simulink model "infeed_base"  (R2023b)
settings: Solver=VariableStepAuto  StartTime=0.0  StopTime=.3  MaxStep=1e-3  RelTol=1e-3  AbsTol=1e-3  EnableMultiTasking=on
values from neighbouring files (symbols this model uses):
  Ts = ts(k)    [example_MW.m]
  Un = 400    [example_MW.m]
undefined symbols (not defined in the file or in its folder): Cz, It1base, Ki_id, Ki_iq, Ki_vdc, Kp_id, Kp_iq, Kp_vdc, Le, Leq, Lk, om, Req, Rz, Tsc, Udc, Vt1base, wtbase, X_R_Le, X_R_Lk
libraries: ee_lib x15, nesl_utility x11, fl_lib x6, eeGeneralControl x4, eeTransforms x3, slpidlib x2, eeAdaptiveController x1, eePwmGeneratorTwoLevel x1, eeSinusoidalMeasurement x1
settings Model: SimulationMode=accelerator  Creator=neugebch  LastModifiedBy=neugebch
settings SolverCC: AutoScaleAbsTol=off  AlgebraicLoopSolver=TrustRegion  MaxZcPerStep=1
settings DataIOCC: LimitDataPoints=on  MaxDataPoints=10000
settings OptimizationCC: ReuseModelBlockBuffer=off  LifeSpan=inf
settings DebuggingCC: UnconnectedInputMsg=warning  UnconnectedOutputMsg=warning  UnconnectedLineMsg=warning  AllowSymbolicDim=off  SFUnexpectedBacktrackingDiag=warning  SFNoUnconditionalDefaultTransitionDiag=warning  SFExecutionAtInitializationDiag=none  ArithmeticOperatorsInVariantConditions=warning
settings ModelReferenceCC: EnableRefExpFcnMdlSchedulingChecks=on
settings SFSimCC: SimUseLocalCustomCode=off  CustomCodeUndefinedFunction=UseInterfaceOnly
settings RTWCC: RTWUseLocalCustomCode=off  DLArmComputeVersion=19.05
settings CodeAppCC: StateflowObjectComments=on
settings GRTTargetCC: TargetLangStandard=C89/C90 (ANSI)
settings ConfigComp: CovMetricSettings=dw  CovSaveCumulativeToWorkspaceVar=on  CovSaveSingleToWorkspaceVar=on  CovExternalEMLEnable=off  CovSFcnEnable=off
settings SimscapeCC: SimscapeLogType=all  SimscapeLogSimulationStatistics=on  SimscapeLogDataHistory=10000

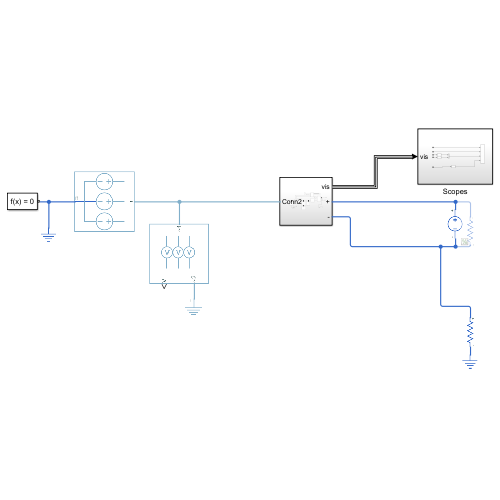
[thumbnail: Simulink's stored preview of the top-level diagram]
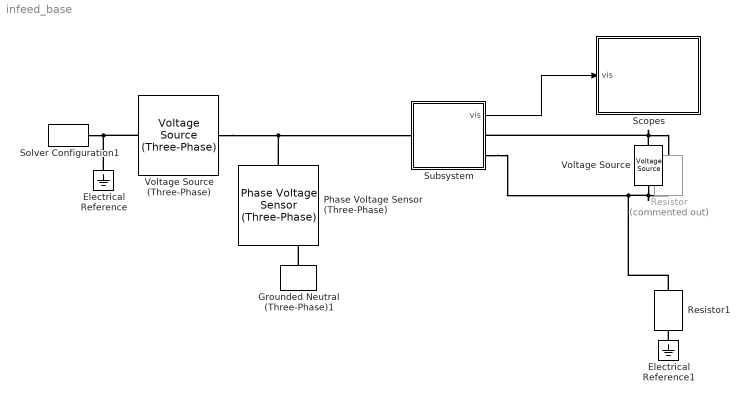
== system infeed_base ==
  Electrical Reference : fl_lib/Electrical/Electrical Elements/Electrical Reference
  Electrical Reference1 : fl_lib/Electrical/Electrical Elements/Electrical Reference
  Grounded Neutral (Three-Phase)1 : ee_lib/Connectors & References/Grounded Neutral (Three-Phase)
  Phase Voltage Sensor (Three-Phase) : ee_lib/Sensors & Transducers/Phase Voltage Sensor (Three-Phase)
  Resistor : fl_lib/Electrical/Electrical Elements/Resistor  Commented=on  R=2 Ohm  i_specify=off  i_priority=None  i=0 A  i_nominal_specify=off  i_nominal_unit=A  i_nominal_value=1  v_specify=off  v_priority=None  v=0 V  v_nominal_specify=off  v_nominal_unit=V  v_nominal_value=1
  Resistor1 : fl_lib/Electrical/Electrical Elements/Resistor  R=1e6 Ohm  i_specify=off  i_priority=None  i=0 A  i_nominal_specify=off  i_nominal_unit=A  i_nominal_value=1  v_specify=off  v_priority=None  v=0 V  v_nominal_specify=off  v_nominal_unit=V  v_nominal_value=1
  Scopes : Subsystem
  Solver Configuration1 : nesl_utility/Solver Configuration  PhysicalDomain=network_engine_domain  SubClassName=solver  LeftPortType=input  RightPortType=generic  Tones=[]  Harmonics=[]  SimulateNoise=off  Profile=off  UseLocalSampling=off  EnableSwitchedLinearOptims=on  FrequencyDomain=off  UseCCode=off  RelTol=0.001  AbsTol=1e-06  MinStep=1e-09  ToWorkspace=off  RevertToSquareIcSolve=off  NumHomotopyIterations=100  PhasorMode=off  PhasorModeNumHarmonics=1  ConsistencySolver=NEWTON_FTOL  IndexReductionMethod=DerivativeReplacement  DoDC=off  ResidualTolerance=1e-09  ConsistencyTolSource=GLOBAL  ConsistencyAbsTol=0.001  ConsistencyRelTol=0.001  ConsistencyTolFactor=0.001  UseLocalSolver=on  LocalSolverChoice=NE_PARTITIONING_ADVANCER  ResolveIndetEquations=on  FunctionEvalNumThread=1  LocalSolverSampleTime=Ts  DoFixedCost=on  MaxNonlinIter=5  MaxModeIter=2  ComputeImpulses=off  ImpulseIterations=1  LinearAlgebra=auto  LinearAlgebraNumThread=0  EquationFormulation=NE_TIME_EF  DelaysMemoryBudget=1024  AutomaticFiltering=on  FilteringTimeConstant=0.001  PartitionStorageMethod=AS_NEEDED  PartitionMemoryBudget=1024  PartitionMethod=ROBUST  MultibodyUseLocalSolver=off  MultibodyLocalSolverChoice=ODE1  MultibodyLocalSolverSampleTime=0.001
  Subsystem : Subsystem
  Voltage Source (Three-Phase) : ee_lib/Sources/Voltage Source (Three-Phase)  vline_rms=sqrt(3) * Un / sqrt(2) V  shift=0 deg  freq=fn Hz  impedance_option=1  SShortCircuit=Skv A*V  XR=X_R  R=0.01 Ohm  L=3.97e-4 H  harmonic_option=1  harmonic_orders=[5, 7, 11, 13]  harmonic_ratios=[.1, .1, .1, .1]  G_parasitic=0 1/Ohm  I_specify=off  I_priority=None  I=[0, 0, 0] A  I_nominal_specify=off  I_nominal_unit=A  I_nominal_value=1
  Voltage Source : ee_lib/Sources/Voltage Source  dc_voltage=Udc V  ac_voltage=0 V  ac_shift=0 rad  ac_frequency=fn Hz  noise_mode=ee.enum.sources.noise.Disabled  PSD=0 V^2/Hz  sample_time=1e-3 s  repeatability=ee.enum.sources.repeatability.NotRepeatable  user_seed=0  auto_seed=3499211588  i_specify=off  i_priority=None  i=0 A  i_nominal_specify=off  i_nominal_unit=A  i_nominal_value=1  v_specify=off  v_priority=None  v=0 V  v_nominal_specify=off  v_nominal_unit=V  v_nominal_value=1
  wires:
  Subsystem/1(vis) -> Scopes/1(vis)
  connections:
  Electrical Reference/LConn1 -- Solver Configuration1/RConn1 -- Voltage Source (Three-Phase)/LConn1
  Grounded Neutral (Three-Phase)1/LConn1 -- Phase Voltage Sensor (Three-Phase)/RConn2
  Voltage Source/RConn1 -- Resistor1/LConn1 -- Subsystem/RConn2 -- Resistor/RConn1
  Electrical Reference1/LConn1 -- Resistor1/RConn1
  Voltage Source/LConn1 -- Subsystem/RConn1 -- Resistor/LConn1
  Voltage Source (Three-Phase)/RConn1 -- Phase Voltage Sensor (Three-Phase)/LConn1 -- Subsystem/LConn1

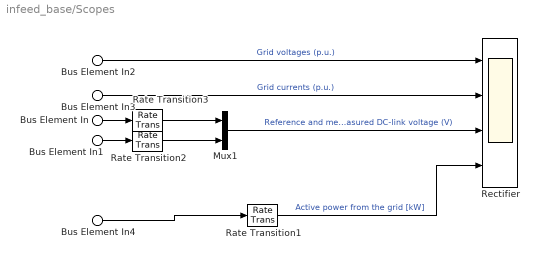
== system infeed_base/Scopes ==
  Bus Element In : Inport  PortName=vis  Element=VdcRef
  Bus Element In1 : Inport  PortName=vis  Element=VdcF
  Bus Element In2 : Inport  PortName=vis  Element=VgABC
  Bus Element In3 : Inport  PortName=vis  Element=IgABC
  Bus Element In4 : Inport  PortName=vis  Element=Pt
  Mux1 : Mux  Inputs=2
  Rate Transition1 : RateTransition
  Rate Transition2 : RateTransition
  Rate Transition3 : RateTransition
  Rectifier : Scope  NumInputPorts=4
  wires:
  Rate Transition2/1 -> Mux1/2
  Bus Element In/1 -> Rate Transition3/1
  Mux1/1 -> Rectifier/3  "Reference and measured DC-link voltage (V)"
  Bus Element In4/1 -> Rate Transition1/1
  Bus Element In2/1 -> Rectifier/1  "Grid voltages (p.u.)"
  Bus Element In3/1 -> Rectifier/2  "Grid currents (p.u.)"
  Rate Transition1/1 -> Rectifier/4  "Active power from the grid [kW]"
  Bus Element In1/1 -> Rate Transition2/1
  Rate Transition3/1 -> Mux1/1

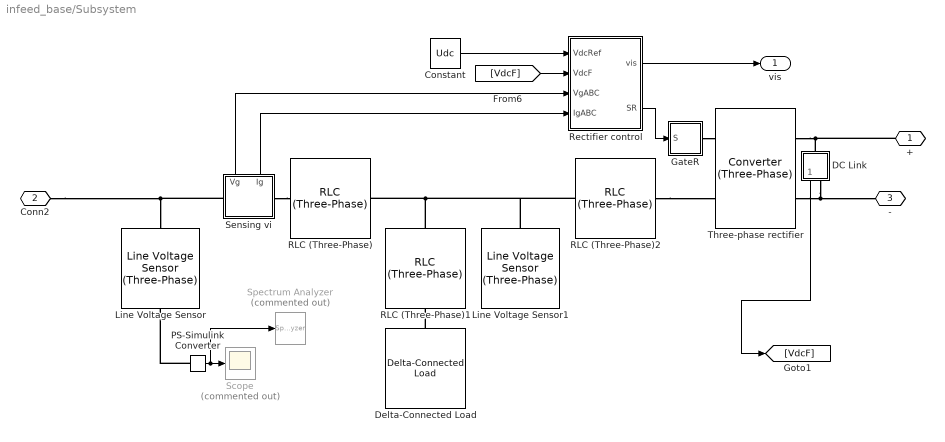
== system infeed_base/Subsystem ==
  Constant : Constant  Value=Udc
  DC Link : Subsystem
  Delta-Connected Load : ee_lib/Passive/RLC Assemblies/Delta-Connected Load  parameterization=ee.enum.rlc.parameterization.direct  component_structure=ee.enum.rlc.structure.C  component_structure_PQ=ee.enum.rlc.structure.SeriesRC  R=1 Ohm  L=1e-3 H  C=Cz F  VRated=24e3 V  FRated=60 Hz  P=1e3 W  Qpos=1e2 A*V  Qneg=-1e2 A*V  R_parasitic=0 Ohm  G_parasitic=0 1/Ohm  R_parasitic_PQ=0 Ohm  G_parasitic_PQ=0 1/Ohm  Vmag0=24e3 V  Vang0=0 deg  Freq0=60 Hz  IL_specify=off  IL_priority=High  IL=[0, 0, 0] A  IL_nominal_specify=off  IL_nominal_unit=A  IL_nominal_value=1  VC_specify=off  VC_priority=High  VC=[0, 0, 0] V  VC_nominal_specify=off  VC_nominal_unit=V  VC_nominal_value=1
      settings: InternalSimscapePortConfiguration="{\"Bottom\":[],\"Left\":[{\"id\":\"N\",\"label\":\"~\",\"type\":\"foundation.electrical.three_phase\"}],\"Right\":[],\"Top\":[]}"
  GateR : Subsystem
  Line Voltage Sensor : ee_lib/Sensors & Transducers/Line Voltage Sensor (Three-Phase)
  Line Voltage Sensor1 : ee_lib/Sensors & Transducers/Line Voltage Sensor (Three-Phase)
  PS-Simulink Converter : nesl_utility/PS-Simulink Converter  PhysicalDomain=network_engine_domain  SubClassName=ps_output  LeftPortType=input  RightPortType=output  PseudoPeriodic=off  Frequencies=[]  VectorFormat=inherit  Unit=inherit  AffineConversion=off
  RLC (Three-Phase) : ee_lib/Passive/RLC Assemblies/RLC (Three-Phase)  component_structure=ee.enum.rlc.structure.SeriesRL  R=Le*om/X_R_Le Ohm  L=Le H  C=1e-6 F  R_parasitic=0 Ohm  G_parasitic=0 1/Ohm  IL_specify=off  IL_priority=High  IL=[0, 0, 0] A  IL_nominal_specify=off  IL_nominal_unit=A  IL_nominal_value=1  VC_specify=off  VC_priority=High  VC=[0, 0, 0] V  VC_nominal_specify=off  VC_nominal_unit=V  VC_nominal_value=1
      settings: InternalSimscapePortConfiguration="{\"Bottom\":[],\"Left\":[{\"id\":\"N1\",\"label\":\"~1\",\"type\":\"foundation.electrical.three_phase\"}],\"Right\":[{\"id\":\"N2\",\"label\":\"~2\",\"type\":\"foundation.electrical.three_phase\"}],\"Top\":[]}"
  RLC (Three-Phase)1 : ee_lib/Passive/RLC Assemblies/RLC (Three-Phase)  component_structure=ee.enum.rlc.structure.R  R=Rz Ohm  L=1e-3 H  C=1e-6 F  R_parasitic=0 Ohm  G_parasitic=0 1/Ohm  IL_specify=off  IL_priority=High  IL=[0, 0, 0] A  IL_nominal_specify=off  IL_nominal_unit=A  IL_nominal_value=1  VC_specify=off  VC_priority=High  VC=[0, 0, 0] V  VC_nominal_specify=off  VC_nominal_unit=V  VC_nominal_value=1
      settings: InternalSimscapePortConfiguration="{\"Bottom\":[],\"Left\":[{\"id\":\"N1\",\"label\":\"~1\",\"type\":\"foundation.electrical.three_phase\"}],\"Right\":[{\"id\":\"N2\",\"label\":\"~2\",\"type\":\"foundation.electrical.three_phase\"}],\"Top\":[]}"
  RLC (Three-Phase)2 : ee_lib/Passive/RLC Assemblies/RLC (Three-Phase)  component_structure=ee.enum.rlc.structure.SeriesRL  R=Lk*om/X_R_Lk Ohm  L=Lk H  C=1e-6 F  R_parasitic=0 Ohm  G_parasitic=0 1/Ohm  IL_specify=off  IL_priority=High  IL=[0, 0, 0] A  IL_nominal_specify=off  IL_nominal_unit=A  IL_nominal_value=1  VC_specify=off  VC_priority=High  VC=[0, 0, 0] V  VC_nominal_specify=off  VC_nominal_unit=V  VC_nominal_value=1
      settings: InternalSimscapePortConfiguration="{\"Bottom\":[],\"Left\":[{\"id\":\"N1\",\"label\":\"~1\",\"type\":\"foundation.electrical.three_phase\"}],\"Right\":[{\"id\":\"N2\",\"label\":\"~2\",\"type\":\"foundation.electrical.three_phase\"}],\"Top\":[]}"
  Rectifier control : Subsystem
  Scope : Scope  Commented=on
  Sensing vi : Subsystem
      settings: PortSchema="{\"entries\":[{\"content\":{\"sides\":[{\"content\":{\"connectorIds\":[\"LConn1\"]},\"type\":\"ConnectorPlacement.EquallySpacedRectSide\",\"uuid\":\"c5057f2e-2c18-4118-b873-a75143a124e4\"},{\"content\":{\"connectorIds\":[\"RConn1\"],\"side\":\"RIGHT\"},\"type\":\"ConnectorPlacement.EquallySpacedRectSide\",\"uuid\":\"847dbac9-66f5-462a-b095-b42c8738b9ce\"},{\"content\":{\"connectorIds\":[\"Out1\",\"Out2\"],\"side\":\"TOP\"},\"type\":\"ConnectorPlacement.EquallySpacedRectSide\",\"uuid\":\"1cd52aa7-c39c-45ef-b799-a348546c5bc9\"}]},\"type\":\"ConnectorPlacement.EquallySpacedConnector\",\"uuid\":\"7d89bf63-b784-4419-8d3e-10ce7abb2518\"}],\"packageUris\":[\"http://schema.mathworks.com/mf0/Connector/R2020b\"],\"version\":\"1.0\"}"
  Spectrum Analyzer : SpectrumAnalyzer  Commented=on  WindowPosition=[1 31 1920 973]  Method=Welch  SampleRate=1000000  PlotAsTwoSidedSpectrum=off  AxesScaling=Manual  Span=500000  CenterFrequency=250000  StartFrequency=0  StopFrequency=500000  RBWSource=Property  RBW=5  Window=Rectangular  AveragingMethod=Exponential  YLimits=[-2.9752431145922511035,92.887308708132081847]
  Three-phase rectifier : ee_lib/Semiconductors & Converters/Converters/Converter (Three-Phase)  port_option=ee.enum.threePhasePort.composite  device_type=ee.enum.converters.switchingdevice.igbt  K=0  Vf=0.8 V  Ron=0.001 Ohm  Rds=0.001 Ohm  Goff=1e-5 1/Ohm  Vgt=1 V  Vgt_off=-1 V  Ih=1 A  Vth=0.5 V  diode_param=ee.enum.converters.protectiondiode.nodynamics  diode_Vf=0.8 V  diode_Ron=0.001 Ohm  diode_Goff=1e-5 1/Ohm  diode_C=50 nF  diode_iRM=-235 A  diode_iF=300 A  diode_idot=-50 A/us  diode_trr_param=ee.enum.converters.diodetrr.trr_factor  diode_trr_factor=3  diode_trr=15 us  diode_Qrr=1.5e+3 s*uA  snubber_type=ee.enum.converters.snubber.exclude  Cs=1e-5 F  Rs=1e-3 Ohm
  + : PMIOPort  Side=Right
  Conn2 : PMIOPort  Port=2  Side=Left
  - : PMIOPort  Port=3  Side=Right
  vis : Outport
  wires:
  Sensing vi/2(Ig) -> Rectifier control/4(IgABC)
  Rectifier control/1(vis) -> vis/1
  PS-Simulink Converter/1 -> Spectrum Analyzer/1, Scope/1
  Sensing vi/1(Vg) -> Rectifier control/3(VgABC)
  [VdcF] -> Rectifier control/2(VdcF)
  Rectifier control/2(SR) -> GateR/1(S)
  Constant/1 -> Rectifier control/1(VdcRef)
  DC Link/1(vdcF) -> [VdcF]
  connections:
  RLC (Three-Phase)1/LConn1 -- Line Voltage Sensor1/LConn1 -- RLC (Three-Phase)2/LConn1 -- RLC (Three-Phase)/RConn1
  PS-Simulink Converter/LConn1 -- Line Voltage Sensor/RConn1
  RLC (Three-Phase)2/RConn1 -- Three-phase rectifier/LConn2
  Sensing vi/LConn1 -- Conn2/RConn1 -- Line Voltage Sensor/LConn1
  Three-phase rectifier/RConn1 -- +/RConn1 -- DC Link/LConn1
  Delta-Connected Load/LConn1 -- RLC (Three-Phase)1/RConn1
  GateR/RConn1 -- Three-phase rectifier/LConn1
  DC Link/RConn1 -- -/RConn1 -- Three-phase rectifier/RConn2
  Sensing vi/RConn1 -- RLC (Three-Phase)/LConn1

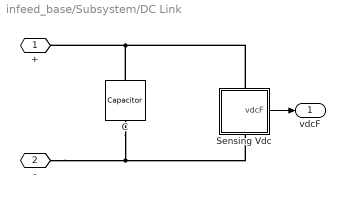
== system infeed_base/Subsystem/DC Link ==
  C : fl_lib/Electrical/Electrical Elements/Capacitor  c=500e-6; F  r=2e-3 Ohm  g=0 1/Ohm  i_specify=off  i_priority=None  i=0 A  i_nominal_specify=off  i_nominal_unit=A  i_nominal_value=1  v_specify=off  v_priority=None  v=0 V  v_nominal_specify=off  v_nominal_unit=V  v_nominal_value=1  vc_specify=on  vc_priority=None  vc=0 V  vc_nominal_specify=off  vc_nominal_unit=V  vc_nominal_value=1
  Sensing Vdc : Subsystem
      settings: PortSchema="{\"entries\":[{\"content\":{\"sides\":[{\"content\":{\"connectorIds\":[\"LConn1\"]},\"type\":\"ConnectorPlacement.EquallySpacedRectSide\",\"uuid\":\"0c76379d-baff-4140-87e0-7680e80a3e64\"},{\"content\":{\"connectorIds\":[\"RConn1\"],\"side\":\"RIGHT\"},\"type\":\"ConnectorPlacement.EquallySpacedRectSide\",\"uuid\":\"435fa78d-19d1-48b9-8f1c-afd8cf746df8\"},{\"content\":{\"connectorIds\":[],\"side\":\"TOP\"},\"type\":\"ConnectorPlacement.EquallySpacedRectSide\",\"uuid\":\"64f7027d-3f1c-43c6-9f97-24bcd914447a\"},{\"content\":{\"connectorIds\":[\"Out1\"],\"side\":\"BOTTOM\"},\"type\":\"ConnectorPlacement.EquallySpacedRectSide\",\"uuid\":\"c8d3e8f7-8819-4adf-938e-d95e3be67703\"}]},\"type\":\"ConnectorPlacement.EquallySpacedConnector\",\"uuid\":\"559fa4aa-2e9f-4f72-acfb-6b72122ee549\"}],\"packageUris\":[\"http://schema.mathworks.com/mf0/Connector/R2020b\"],\"version\":\"1.0\"}"
  + : PMIOPort  Side=Left
  - : PMIOPort  Port=2  Side=Right
  vdcF : Outport
  wires:
  Sensing Vdc/1(vdcF) -> vdcF/1
  connections:
  -/RConn1 -- C/RConn1 -- Sensing Vdc/RConn1
  C/LConn1 -- Sensing Vdc/LConn1 -- +/RConn1

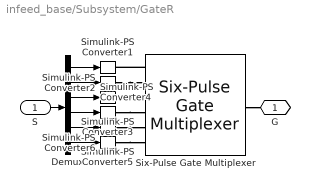
== system infeed_base/Subsystem/GateR ==
  S : Inport
  Demux : Demux  Outputs=6
  Simulink-PS Converter{1..6} (6 alike) : nesl_utility/Simulink-PS Converter  PhysicalDomain=network_engine_domain  SubClassName=ps_input  LeftPortType=input  RightPortType=output  PseudoPeriodic=off  Frequencies=[]  NoiseDistribution=none  NoiseParameters=[]  Unit=1  AffineConversion=off  FilteringAndDerivatives=zero  SimscapeFilterOrder=1  InputFilterTimeConstant=0.001  UdotUserProvided=1
  Six-Pulse Gate Multiplexer : ee_lib/Semiconductors & Converters/Converters/Six-Pulse Gate Multiplexer  port_option=ee.enum.controlport.ps
  G : PMIOPort  Side=Right
  wires:
  Demux/4 -> Simulink-PS Converter4/1
  Demux/1 -> Simulink-PS Converter1/1
  Demux/2 -> Simulink-PS Converter2/1
  S/1 -> Demux/1
  Demux/5 -> Simulink-PS Converter5/1
  Demux/6 -> Simulink-PS Converter6/1
  Demux/3 -> Simulink-PS Converter3/1
  connections:
  Simulink-PS Converter4/RConn1 -- Six-Pulse Gate Multiplexer/LConn4
  Simulink-PS Converter2/RConn1 -- Six-Pulse Gate Multiplexer/LConn2
  Simulink-PS Converter3/RConn1 -- Six-Pulse Gate Multiplexer/LConn3
  Simulink-PS Converter6/RConn1 -- Six-Pulse Gate Multiplexer/LConn6
  Simulink-PS Converter5/RConn1 -- Six-Pulse Gate Multiplexer/LConn5
  Six-Pulse Gate Multiplexer/LConn1 -- Simulink-PS Converter1/RConn1
  Six-Pulse Gate Multiplexer/RConn1 -- G/RConn1

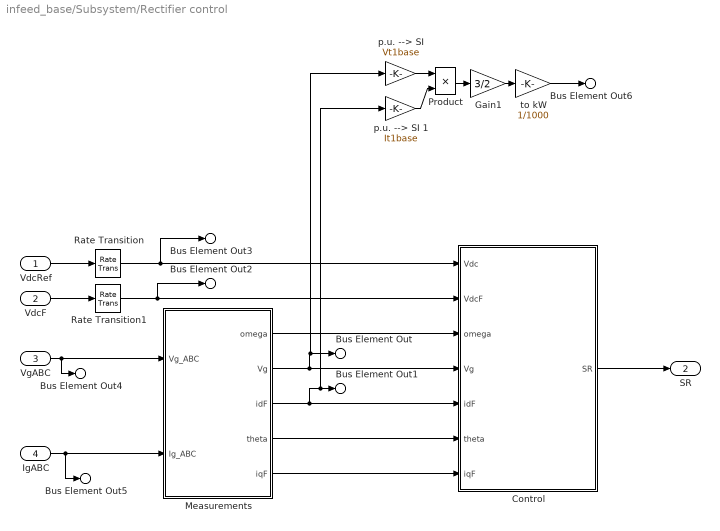
== system infeed_base/Subsystem/Rectifier control ==
  VdcRef : Inport
  VdcF : Inport  Port=2
  VgABC : Inport  Port=3
  IgABC : Inport  Port=4
  Control : Subsystem
  Gain1 : Gain  Gain=3/2
  Measurements : Subsystem
  Product : Product
  Rate Transition : RateTransition
  Rate Transition1 : RateTransition
  p.u. --> SI : Gain  Gain=Vt1base
  p.u. --> SI 1 : Gain  Gain=It1base
  to kW : Gain  Gain=1/1000
  Bus Element Out : Outport  PortName=vis  Element=Vg
  Bus Element Out1 : Outport  PortName=vis  Element=idF
  Bus Element Out2 : Outport  PortName=vis  Element=VdcF
  Bus Element Out3 : Outport  PortName=vis  Element=VdcRef
  Bus Element Out4 : Outport  PortName=vis  Element=VgABC
  Bus Element Out5 : Outport  PortName=vis  Element=IgABC
  Bus Element Out6 : Outport  PortName=vis  Element=Pt
  SR : Outport  Port=2  VectorParamsAs1DForOutWhenUnconnected=off
  wires:
  VdcRef/1 -> Rate Transition/1
  VdcF/1 -> Rate Transition1/1
  VgABC/1 -> Bus Element Out4/1, Measurements/1(Vg_ABC)
  IgABC/1 -> Bus Element Out5/1, Measurements/2(Ig_ABC)
  Measurements/1(omega) -> Control/3(omega)
  Measurements/4(theta) -> Control/6(theta)
  Measurements/5(iqF) -> Control/7(iqF)
  Control/1(SR) -> SR/1
  Rate Transition/1 -> Bus Element Out3/1, Control/1(Vdc)
  Rate Transition1/1 -> Bus Element Out2/1, Control/2(VdcF)
  Measurements/2(Vg) -> p.u. --> SI/1, Bus Element Out/1, Control/4(Vg)
  p.u. --> SI 1/1 -> Product/2
  p.u. --> SI/1 -> Product/1
  Gain1/1 -> to kW/1
  Product/1 -> Gain1/1
  Measurements/3(idF) -> p.u. --> SI 1/1, Bus Element Out1/1, Control/5(idF)
  to kW/1 -> Bus Element Out6/1

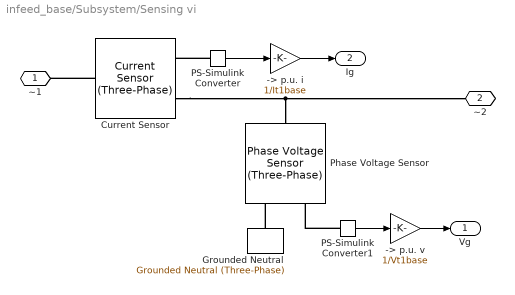
== system infeed_base/Subsystem/Sensing vi ==
  -> p.u. i : Gain  Gain=1/It1base
  -> p.u. v : Gain  Gain=1/Vt1base
  Current Sensor : ee_lib/Sensors & Transducers/Current Sensor (Three-Phase)
  Grounded Neutral : ee_lib/Connectors & References/Grounded Neutral (Three-Phase)
  PS-Simulink Converter : nesl_utility/PS-Simulink Converter  PhysicalDomain=network_engine_domain  SubClassName=ps_output  LeftPortType=input  RightPortType=output  PseudoPeriodic=off  Frequencies=[]  VectorFormat=1-D array  Unit=1  AffineConversion=off
  PS-Simulink Converter1 : nesl_utility/PS-Simulink Converter  PhysicalDomain=network_engine_domain  SubClassName=ps_output  LeftPortType=input  RightPortType=output  PseudoPeriodic=off  Frequencies=[]  VectorFormat=1-D array  Unit=1  AffineConversion=off
  Phase Voltage Sensor : ee_lib/Sensors & Transducers/Phase Voltage Sensor (Three-Phase)
  ~1 : PMIOPort  Side=Left
  ~2 : PMIOPort  Port=2  Side=Right
  Vg : Outport
  Ig : Outport  Port=2
  wires:
  -> p.u. i/1 -> Ig/1
  PS-Simulink Converter1/1 -> -> p.u. v/1
  PS-Simulink Converter/1 -> -> p.u. i/1
  -> p.u. v/1 -> Vg/1
  connections:
  PS-Simulink Converter1/LConn1 -- Phase Voltage Sensor/RConn1
  Current Sensor/RConn2 -- Phase Voltage Sensor/LConn1 -- ~2/RConn1
  PS-Simulink Converter/LConn1 -- Current Sensor/RConn1
  Grounded Neutral/LConn1 -- Phase Voltage Sensor/RConn2
  Current Sensor/LConn1 -- ~1/RConn1

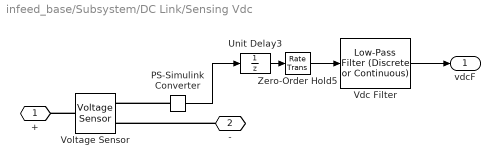
== system infeed_base/Subsystem/DC Link/Sensing Vdc ==
  PS-Simulink Converter : nesl_utility/PS-Simulink Converter  PhysicalDomain=network_engine_domain  SubClassName=ps_output  LeftPortType=input  RightPortType=output  PseudoPeriodic=off  Frequencies=[]  VectorFormat=1-D array  Unit=1  AffineConversion=off
  Unit Delay3 : UnitDelay  SampleTime=Ts  HasFrameUpgradeWarning=on
  Vdc Filter : eeGeneralControl/Low-Pass Filter (Discrete or Continuous)  K=1  T=1e-3  B=inf  A=-inf  init_option=Inherited from block input  x0=0  Ts=Tsc
  Voltage Sensor : fl_lib/Electrical/Electrical Sensors/Voltage Sensor
  Zero-Order Hold5 : RateTransition  OutPortSampleTime=5e-05
  + : PMIOPort  Side=Left
  - : PMIOPort  Port=2  Side=Right
  vdcF : Outport
  wires:
  Unit Delay3/1 -> Zero-Order Hold5/1
  Zero-Order Hold5/1 -> Vdc Filter/1
  Vdc Filter/1 -> vdcF/1
  PS-Simulink Converter/1 -> Unit Delay3/1
  connections:
  -/RConn1 -- Voltage Sensor/RConn2
  Voltage Sensor/LConn1 -- +/RConn1
  PS-Simulink Converter/LConn1 -- Voltage Sensor/RConn1

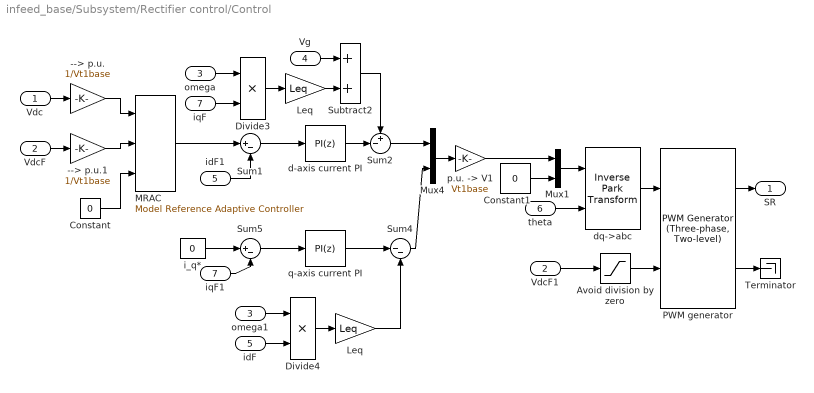
== system infeed_base/Subsystem/Rectifier control/Control ==
  Vdc : Inport
  VdcF : Inport  Port=2
  omega : Inport  Port=3
  Vg : Inport  Port=4
  idF : Inport  Port=5
  theta : Inport  Port=6
  iqF : Inport  Port=7
  --> p.u. : Gain  Gain=1/Vt1base
  --> p.u.1 : Gain  Gain=1/Vt1base
  Avoid division by zero : Saturate  UpperLimit=1e6  LowerLimit=10
  Constant : Constant  Value=0
  Constant1 : Constant  Value=0  SampleTime=Tsc
  Divide3 : Product  Inputs=**
  Divide4 : Product  Inputs=**
  Leq : Gain  Gain=Leq
  "Leq " : Gain  Gain=Leq
  MRAC : eeAdaptiveController/Model Reference Adaptive Controller  Kp=Kp_vdc  Ki=Ki_vdc  Kd=0  Kaw=1000  UseFilter=off  N=100  up=5  lo=-5  Ts=Tsc  TfType=Discrete-time  numd=numd  dend=dend  numc=[1 1]  denc=[1 2 1]  Tsd=0.01  gamma=0.8
  Mux1 : Mux  Inputs=2
  Mux4 : Mux  Inputs=2
  PWM generator : eePwmGeneratorTwoLevel/PWM Generator (Three-phase, Two-level)  PWMMode=Continuous PWM (CPWM)  CPWMMode=SVM: space vector modulation  DPWMMode=60 DPWM: 60 degree discontinuous PWM  fsw=fsw  Ts=Ts
  Subtract2 : Sum
  Sum1 : Sum  Inputs=|+-
  Sum2 : Sum  Inputs=+-|
  Sum4 : Sum  Inputs=|--
  Sum5 : Sum  Inputs=|+-
  Terminator : Terminator
  VdcF1 : InportShadow  Port=2
  d-axis current PI : slpidlib/PID Controller  Controller=PI  Form=Parallel  TimeDomain=Discrete-time  UseExternalTs=off  SampleTime=Tsc  IntegratorMethod=Forward Euler  FilterMethod=Forward Euler  ControllerParametersSource=internal  P=Kp_id  I=Ki_id  UseKiTs=off  D=0  N=100  UseFilter=on  TunerSelectOption=Transfer Function Based (PID Tuner App)  InitialConditionSource=internal  InitialConditionForIntegrator=0  InitialConditionForFilter=0  DifferentiatorICPrevScaledInput=0  ExternalReset=none  TrackingMode=off  Kt=1  LimitOutput=on  SatLimitsSource=internal  UpperSaturationLimit=Req*1*10  LowerSaturationLimit=-Req*1*10  LinearizeAsGain=on  AntiWindupMode=back-calculation  Kb=1000  LimitIntegrator=off  UpperIntegratorSaturationLimit=inf  LowerIntegratorSaturationLimit=-inf  POutMin=[]  POutMax=[]  IOutMin=[]  IOutMax=[]  DOutMin=[]  DOutMax=[]  NOutMin=[]  NOutMax=[]  SumOutMin=[]  SumOutMax=[]  SaturationOutMin=[]  SaturationOutMax=[]  PParamMin=[]  PParamMax=[]  IParamMin=[]  IParamMax=[]  DParamMin=[]  DParamMax=[]  NParamMin=[]  NParamMax=[]  KbParamMin=[]  KbParamMax=[]  KtParamMin=[]  KtParamMax=[]  KbOutMin=[]  KbOutMax=[]  KtOutMin=[]  KtOutMax=[]  IntegratorOutMin=[]  IntegratorOutMax=[]  FilterOutMin=[]  FilterOutMax=[]  SumI1OutMin=[]  SumI1OutMax=[]  SumI2OutMin=[]  SumI2OutMax=[]  SumI3OutMin=[]  SumI3OutMax=[]  SumI4OutMin=[]  SumI4OutMax=[]  SumDOutMin=[]  SumDOutMax=[]  DifferentiatorOutMin=[]  DifferentiatorOutMax=[]  FilterDiffOutCoefMin=[]  FilterDiffOutCoefMax=[]  ReciprocalOutMin=[]  ReciprocalOutMax=[]  SumDenOutMin=[]  SumDenOutMax=[]  SumNumOutMin=[]  SumNumOutMax=[]  DivideOutMin=[]  DivideOutMax=[]  UdiffTsProdOutMin=[]  UdiffTsProdOutMax=[]  NTsProdOutMin=[]  NTsProdOutMax=[]  UintegralTsProdOutMin=[]  UintegralTsProdOutMax=[]  UngainTsProdOutMin=[]  UngainTsProdOutMax=[]  ClampingZeroOutDataTypeStr=Inherit: Inherit via back propagation  ClampingZeroOutMin=[]  ClampingZeroOutMax=[]  FilterDenConstantOutDataTypeStr=Inherit: Inherit via back propagation  FilterDenConstantOutMin=[]  FilterDenConstantOutMax=[]  PCopyOutDataTypeStr=Inherit: Inherit via back propagation  PCopyOutMin=[]  PCopyOutMax=[]  NCopyOutDataTypeStr=Inherit: Inherit via back propagation  NCopyOutMin=[]  NCopyOutMax=[]  IntegratorContinuousStateAttributes=''  IntegratorStateMustResolveToSignalObject=off  IntegratorRTWStateStorageClass=Auto  FilterContinuousStateAttributes=''  FilterStateMustResolveToSignalObject=off  FilterRTWStateStorageClass=Auto  ParallelPVariant=InternalParameters  IdealPVariant=Disabled  IVariant=InternalParameters  DVariant=Disabled  IntegratorVariant=Discrete  SatVariant=Enabled  AWVariant=BackCalculation  PCopyVariant=Disabled  TRVariant=Disabled  FdbkBlocksVariant=Forward  IdealPFdbkVariant=Disabled  SatFdbkVariant=Disabled  DerivativeFilterVariant=Disabled  NVariant=Disabled  NCopyVariant=Disabled_SignalSpec  FilterICVariant=Disabled  IntegratorICVariant=InternalICs  ExternalResetVariant=Disabled  TRSumVariant=Passthrough  SumFdbkVariant=Disabled  SumVariant=Sum_PI  TsampFilterVariant=InternalTs  TsampNgainVariant=Passthrough  TsampIntegralVariant=Disabled_SignalSpec  ExternalSaturationOutDataTypeStr=Inherit: Same as second input
  dq->abc : eeTransforms/Inverse Park Transform  AxisAlignment=Q-axis  PowerInvariant=off
  i_q* : Constant  Value=0
  idF1 : InportShadow  Port=5
  iqF1 : InportShadow  Port=7
  omega1 : InportShadow  Port=3
  "p.u. -> V1" : Gain  Gain=Vt1base
  q-axis current PI : slpidlib/PID Controller  Controller=PI  Form=Parallel  TimeDomain=Discrete-time  UseExternalTs=off  SampleTime=Tsc  IntegratorMethod=Forward Euler  FilterMethod=Forward Euler  ControllerParametersSource=internal  P=Kp_iq  I=Ki_iq  UseKiTs=off  D=0  N=100  UseFilter=on  TunerSelectOption=Transfer Function Based (PID Tuner App)  InitialConditionSource=internal  InitialConditionForIntegrator=0  InitialConditionForFilter=0  DifferentiatorICPrevScaledInput=0  ExternalReset=none  TrackingMode=off  Kt=1  LimitOutput=on  SatLimitsSource=internal  UpperSaturationLimit=Req*1*10  LowerSaturationLimit=-Req*1*10  LinearizeAsGain=on  AntiWindupMode=back-calculation  Kb=1000  LimitIntegrator=off  UpperIntegratorSaturationLimit=inf  LowerIntegratorSaturationLimit=-inf  POutMin=[]  POutMax=[]  IOutMin=[]  IOutMax=[]  DOutMin=[]  DOutMax=[]  NOutMin=[]  NOutMax=[]  SumOutMin=[]  SumOutMax=[]  SaturationOutMin=[]  SaturationOutMax=[]  PParamMin=[]  PParamMax=[]  IParamMin=[]  IParamMax=[]  DParamMin=[]  DParamMax=[]  NParamMin=[]  NParamMax=[]  KbParamMin=[]  KbParamMax=[]  KtParamMin=[]  KtParamMax=[]  KbOutMin=[]  KbOutMax=[]  KtOutMin=[]  KtOutMax=[]  IntegratorOutMin=[]  IntegratorOutMax=[]  FilterOutMin=[]  FilterOutMax=[]  SumI1OutMin=[]  SumI1OutMax=[]  SumI2OutMin=[]  SumI2OutMax=[]  SumI3OutMin=[]  SumI3OutMax=[]  SumI4OutMin=[]  SumI4OutMax=[]  SumDOutMin=[]  SumDOutMax=[]  DifferentiatorOutMin=[]  DifferentiatorOutMax=[]  FilterDiffOutCoefMin=[]  FilterDiffOutCoefMax=[]  ReciprocalOutMin=[]  ReciprocalOutMax=[]  SumDenOutMin=[]  SumDenOutMax=[]  SumNumOutMin=[]  SumNumOutMax=[]  DivideOutMin=[]  DivideOutMax=[]  UdiffTsProdOutMin=[]  UdiffTsProdOutMax=[]  NTsProdOutMin=[]  NTsProdOutMax=[]  UintegralTsProdOutMin=[]  UintegralTsProdOutMax=[]  UngainTsProdOutMin=[]  UngainTsProdOutMax=[]  ClampingZeroOutDataTypeStr=Inherit: Inherit via back propagation  ClampingZeroOutMin=[]  ClampingZeroOutMax=[]  FilterDenConstantOutDataTypeStr=Inherit: Inherit via back propagation  FilterDenConstantOutMin=[]  FilterDenConstantOutMax=[]  PCopyOutDataTypeStr=Inherit: Inherit via back propagation  PCopyOutMin=[]  PCopyOutMax=[]  NCopyOutDataTypeStr=Inherit: Inherit via back propagation  NCopyOutMin=[]  NCopyOutMax=[]  IntegratorContinuousStateAttributes=''  IntegratorStateMustResolveToSignalObject=off  IntegratorRTWStateStorageClass=Auto  FilterContinuousStateAttributes=''  FilterStateMustResolveToSignalObject=off  FilterRTWStateStorageClass=Auto  ParallelPVariant=InternalParameters  IdealPVariant=Disabled  IVariant=InternalParameters  DVariant=Disabled  IntegratorVariant=Discrete  SatVariant=Enabled  AWVariant=BackCalculation  PCopyVariant=Disabled  TRVariant=Disabled  FdbkBlocksVariant=Forward  IdealPFdbkVariant=Disabled  SatFdbkVariant=Disabled  DerivativeFilterVariant=Disabled  NVariant=Disabled  NCopyVariant=Disabled_SignalSpec  FilterICVariant=Disabled  IntegratorICVariant=InternalICs  ExternalResetVariant=Disabled  TRSumVariant=Passthrough  SumFdbkVariant=Disabled  SumVariant=Sum_PI  TsampFilterVariant=InternalTs  TsampNgainVariant=Passthrough  TsampIntegralVariant=Disabled_SignalSpec  ExternalSaturationOutDataTypeStr=Inherit: Same as second input
  SR : Outport  VectorParamsAs1DForOutWhenUnconnected=off
  wires:
  Sum5/1 -> q-axis current PI/1
  theta/1 -> dq->abc/2
  Sum4/1 -> Mux4/2
  Subtract2/1 -> Sum2/1
  Sum2/1 -> Mux4/1
  Sum1/1 -> d-axis current PI/1
  Avoid division by zero/1 -> PWM generator/2
  Divide4/1 -> "Leq "/1
  Leq/1 -> Subtract2/2
  i_q*/1 -> Sum5/1
  PWM generator/1 -> SR/1
  omega/1 -> Divide3/1
  q-axis current PI/1 -> Sum4/1
  Mux4/1 -> "p.u. -> V1"/1
  Divide3/1 -> Leq/1
  Mux1/1 -> dq->abc/1
  Constant1/1 -> Mux1/2
  "Leq "/1 -> Sum4/2
  idF/1 -> Divide4/2
  PWM generator/2 -> Terminator/1
  dq->abc/1 -> PWM generator/1
  "p.u. -> V1"/1 -> Mux1/1
  iqF/1 -> Divide3/2
  Vg/1 -> Subtract2/1
  iqF1/1 -> Sum5/2
  omega1/1 -> Divide4/1
  idF1/1 -> Sum1/2
  VdcF1/1 -> Avoid division by zero/1
  Vdc/1 -> --> p.u./1
  --> p.u./1 -> MRAC/1
  VdcF/1 -> --> p.u.1/1
  --> p.u.1/1 -> MRAC/2
  Constant/1 -> MRAC/3
  MRAC/1 -> Sum1/1
  d-axis current PI/1 -> Sum2/2

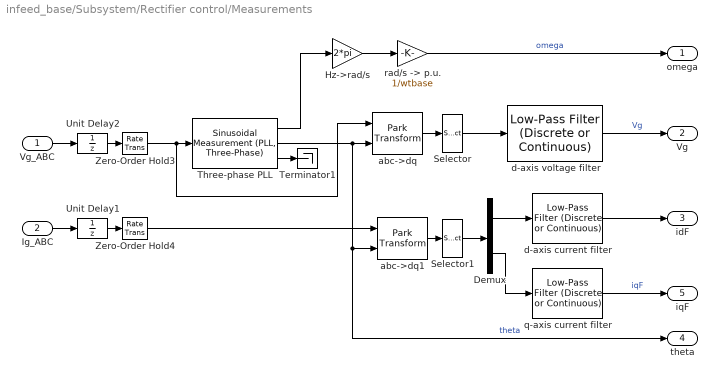
== system infeed_base/Subsystem/Rectifier control/Measurements ==
  Vg_ABC : Inport
  Ig_ABC : Inport  Port=2
  Demux : Demux  Outputs=2
  Hz->rad/s : Gain  Gain=2*pi
  Selector : Selector  InputPortWidth=3  IndexOptions=Index vector (dialog)  Indices=[1]  OutputSizes=1
  Selector1 : Selector  InputPortWidth=3  IndexOptions=Index vector (dialog)  Indices=[1 2]  OutputSizes=1
  Terminator1 : Terminator
  Three-phase PLL : eeSinusoidalMeasurement/Sinusoidal Measurement (PLL, Three-Phase)  Kp_LF=45  Ki_LF=1250  F0=fn  Theta0=0  Ts=Tsc
  Unit Delay1 : UnitDelay  SampleTime=Ts  HasFrameUpgradeWarning=on
  Unit Delay2 : UnitDelay  SampleTime=Ts  HasFrameUpgradeWarning=on
  Zero-Order Hold3 : RateTransition  OutPortSampleTime=5e-05
  Zero-Order Hold4 : RateTransition  OutPortSampleTime=5e-05
  abc->dq : eeTransforms/Park Transform  AxisAlignment=Q-axis  PowerInvariant=off
  abc->dq1 : eeTransforms/Park Transform  AxisAlignment=Q-axis  PowerInvariant=off
  d-axis current filter : eeGeneralControl/Low-Pass Filter (Discrete or Continuous)  K=1  T=1e-3  B=inf  A=-inf  init_option=Inherited from block input  x0=0  Ts=Tsc
  d-axis voltage filter : eeGeneralControl/Low-Pass Filter (Discrete or Continuous)  K=1  T=1e-3  B=inf  A=-inf  init_option=Inherited from block input  x0=0  Ts=Tsc
  q-axis current filter : eeGeneralControl/Low-Pass Filter (Discrete or Continuous)  K=1  T=1e-3  B=inf  A=-inf  init_option=Inherited from block input  x0=0  Ts=Tsc
  "rad/s -> p.u." : Gain  Gain=1/wtbase
  omega : Outport  VectorParamsAs1DForOutWhenUnconnected=off
  Vg : Outport  Port=2  VectorParamsAs1DForOutWhenUnconnected=off
  idF : Outport  Port=3  VectorParamsAs1DForOutWhenUnconnected=off
  theta : Outport  Port=4  VectorParamsAs1DForOutWhenUnconnected=off
  iqF : Outport  Port=5  VectorParamsAs1DForOutWhenUnconnected=off
  wires:
  Unit Delay1/1 -> Zero-Order Hold4/1
  abc->dq/1 -> Selector/1
  Hz->rad/s/1 -> "rad/s -> p.u."/1
  Three-phase PLL/2 -> abc->dq1/2, theta/1, abc->dq/2  "theta"
  d-axis current filter/1 -> idF/1
  Zero-Order Hold3/1 -> abc->dq/1, Three-phase PLL/1
  Three-phase PLL/1 -> Hz->rad/s/1
  Selector/1 -> d-axis voltage filter/1
  Three-phase PLL/3 -> Terminator1/1
  Ig_ABC/1 -> Unit Delay1/1
  d-axis voltage filter/1 -> Vg/1  "Vg"
  Zero-Order Hold4/1 -> abc->dq1/1
  Unit Delay2/1 -> Zero-Order Hold3/1
  Demux/1 -> d-axis current filter/1
  abc->dq1/1 -> Selector1/1
  Selector1/1 -> Demux/1
  Vg_ABC/1 -> Unit Delay2/1
  Demux/2 -> q-axis current filter/1
  "rad/s -> p.u."/1 -> omega/1  "omega"
  q-axis current filter/1 -> iqF/1  "iqF"
